simulink model "SlewAndControlConstrained_Controller_unit_test"  (R2018b)
settings: Solver=VariableStepAuto  StartTime=0.0  StopTime=50  RelTol=1e-3
undefined symbols (not defined in the file or in its folder): fswParams, satelliteDynamics_lib, simParams
libraries: SlewAndControlConstrained_Controller_lib x1, vrlib x1, aerolibutil x1
settings Model: Creator=colem  LastModifiedBy=taylorreynolds

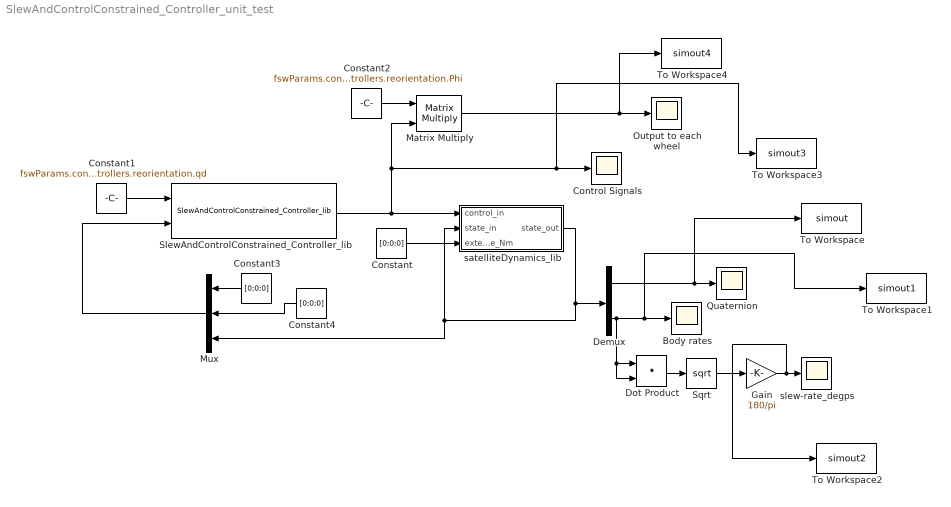
== system SlewAndControlConstrained_Controller_unit_test ==
  Body rates : Scope
  Constant : Constant  Value=[0;0;0]
  Constant1 : Constant  Value=fswParams.controllers.reorientation.qd
  Constant2 : Constant  Value=fswParams.controllers.reorientation.Phi
  Constant3 : Constant  Value=[0;0;0]
  Constant4 : Constant  Value=[0;0;0]
  Control Signals : Scope
  Demux : Demux  Outputs=[4 3]
  Dot Product : DotProduct  InputSameDT=on  OutDataTypeStr=Inherit: Inherit via internal rule
  Gain : Gain  Gain=180/pi
  Matrix Multiply : Product  Multiplication=Matrix(*)
  Mux : Mux  Inputs=[3 3 7]
  Output to each wheel : Scope
  Quaternion : Scope
  SlewAndControlConstrained_Controller_lib : SlewAndControlConstrained_Controller_lib/SlewAndControlConstrained_Controller_lib  SystemSampleTime=-1
  Sqrt : Sqrt  SaturateOnIntegerOverflow=on
  To Workspace : ToWorkspace  VariableName=simout  SaveFormat=Timeseries  SampleTime=-1
  To Workspace1 : ToWorkspace  VariableName=simout1  SaveFormat=Timeseries  SampleTime=-1
  To Workspace2 : ToWorkspace  VariableName=simout2  SaveFormat=Timeseries  SampleTime=-1
  To Workspace3 : ToWorkspace  VariableName=simout3  SaveFormat=Timeseries  SampleTime=-1
  To Workspace4 : ToWorkspace  VariableName=simout4  SaveFormat=Timeseries  SampleTime=-1
  satelliteDynamics_lib : Subsystem  AncestorBlock=satelliteDynamics_lib/satelliteDynamics_lib
  slew-rate_degps : Scope
  wires:
  SlewAndControlConstrained_Controller_lib/1 -> Matrix Multiply/2, To Workspace3/1, Control Signals/1, satelliteDynamics_lib/1(control_in)
  Demux/1 -> To Workspace/1, Quaternion/1
  Demux/2 -> To Workspace1/1, Body rates/1, Dot Product/2, Dot Product/1
  Constant/1 -> satelliteDynamics_lib/3(external_torque_Nm)
  Constant1/1 -> SlewAndControlConstrained_Controller_lib/1
  Constant2/1 -> Matrix Multiply/1
  Matrix Multiply/1 -> To Workspace4/1, Output to each wheel/1
  satelliteDynamics_lib/1(state_out) -> Mux/3, satelliteDynamics_lib/2(state_in), Demux/1
  Constant3/1 -> Mux/1
  Constant4/1 -> Mux/2
  Mux/1 -> SlewAndControlConstrained_Controller_lib/2
  Sqrt/1 -> Gain/1
  Dot Product/1 -> Sqrt/1
  Gain/1 -> To Workspace2/1, slew-rate_degps/1

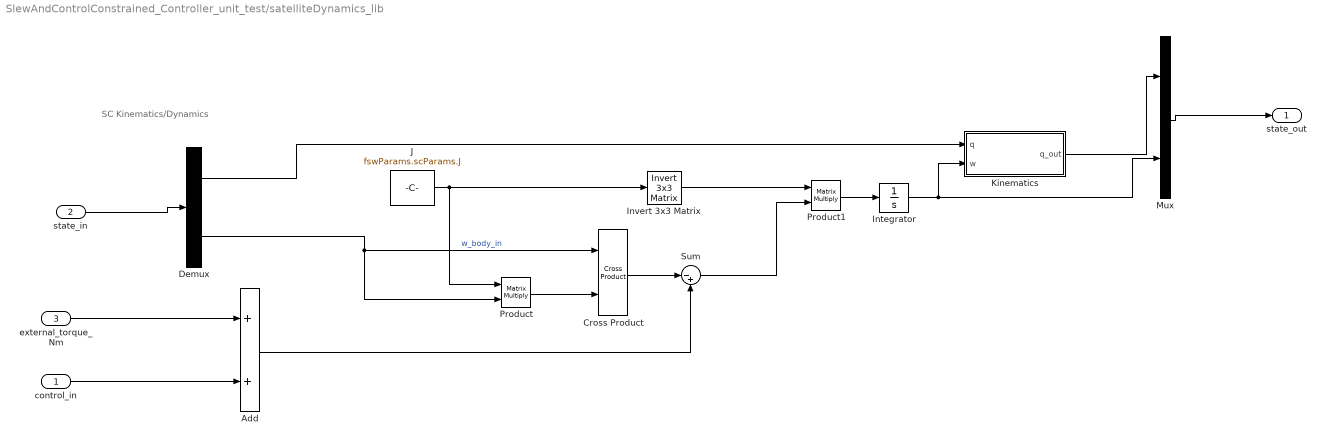
== system SlewAndControlConstrained_Controller_unit_test/satelliteDynamics_lib ==
  note: SC Kinematics/Dynamics
  control_in : Inport
  state_in : Inport  Port=2
  external_torque_Nm : Inport  Port=3
  Add : Sum
  Cross Product : vrlib/Utilities/Cross Product
      settings: SourceProductBaseCode=VR
  Demux : Demux  Outputs=[4 3]
  Integrator : Integrator  InitialCondition=simParams.initialConditions.w0
  Invert 3x3 Matrix : aerolibutil/Invert  3x3 Matrix
  J : Constant  Value=fswParams.scParams.J
  Kinematics : Subsystem
  Mux : Mux  Inputs=[4 3]
  Product : Product  Multiplication=Matrix(*)
  Product1 : Product  Multiplication=Matrix(*)
  Sum : Sum  Inputs=|-+
  state_out : Outport
  wires:
  J/1 -> Product/1, Invert 3x3 Matrix/1
  Product/1 -> Cross Product/2
  Cross Product/1 -> Sum/1
  Sum/1 -> Product1/2
  Invert 3x3 Matrix/1 -> Product1/1
  Product1/1 -> Integrator/1
  Integrator/1 -> Mux/2, Kinematics/2(w)
  Kinematics/1(q_out) -> Mux/1
  Demux/2 -> Cross Product/1, Product/2  "w_body_in"
  Demux/1 -> Kinematics/1(q)
  Mux/1 -> state_out/1
  state_in/1 -> Demux/1
  external_torque_Nm/1 -> Add/1
  control_in/1 -> Add/2
  Add/1 -> Sum/2

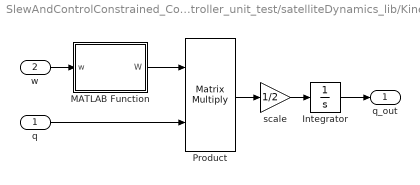
== system SlewAndControlConstrained_Controller_unit_test/satelliteDynamics_lib/Kinematics ==
  q : Inport
  w : Inport  Port=2
  Integrator : Integrator  InitialCondition=simParams.initialConditions.q0
  MATLAB Function : MATLAB Function  TreatAsAtomicUnit=on
  Product : Product  Multiplication=Matrix(*)
  scale : Gain  Gain=1/2
  q_out : Outport
  wires:
  w/1 -> MATLAB Function/1(w)
  MATLAB Function/1(W) -> Product/1
  q/1 -> Product/2
  Product/1 -> scale/1
  scale/1 -> Integrator/1
  Integrator/1 -> q_out/1

== matlab function SlewAndControlConstrained_Controller_unit_test/satelliteDynamics_lib/Kinematics/MATLAB Function ==
  data: w input; W output
function W = fcn(w)
%#codegen

W = [0, -w(1),-w(2),-w(3); w(1), 0,w(3), -w(2); w(2), -w(3), 0, w(1); w(3), w(2), -w(1), 0 ];

end
